simulink model "IEEE123_4subsystem"  (R2022b)
settings: Solver=ode4  StartTime=0.0  StopTime=inf  FixedStep=Ts  MaxStep=1e-4  RelTol=1e-3
PreLoadFcn:
  | Ts = 50e-6;
PostLoadFcn:
  | Ts = 50e-6;
InitFcn:
  | %%%%%%%%%%%%%%%%%%%%%%%%
  | % Simulation data for the IEEE 123 Node Test Feeder model
  | %%%%%%%%%%%%%%%%%%%%%%%
  | 
  | % miles/km
  | mi2km = 1.60934;
  | 
  | % feet to km
  | ft2km = 0.0003048;
  | 
  | % microsiemens to Farads
  | ms2F = 1/2/pi/60*1e-6;
  | 
  | %% Configuration 1 - series reactance - ohm/mile
  | 
  | R_1 = [0.4576 0.1560 0.1535;0.1560 0.4666 0.1580;0.1535 0.1580 0.4615];
  | X_1 = [1.0780 0.5017 0.3849;0.5017 1.0482 0.4236;0.3849 0.4236 1.0651];
  | 
  | % charging susceptance - microsiemens/mile
  | 
  | B_1 = [5.6765 -1.8319 -0.6982;-1.8319 5.9809 -1.1645;-0.6982 -1.1645 5.3971];
  | 
  | % convert for SPS
  | 
  | R_1 = R_1/mi2km;
  | 
  | Rs_1=(R_1(1,1)+R_1(2,2)+R_1(3,3))/3;
  | Rm_1=(R_1(1,2)+R_1(1,3)+R_1(2,3))/3;
  | R1_1=Rs_1-Rm_1;
  | R0_1=Rs_1+2*Rm_1;
  | 
  | L_1 = X_1/mi2km/2/pi/60;
  | 
  | Ls_1=(L_1(1,1)+L_1(2,2)+L_1(3,3))/3;
  | Lm_1=(L_1(1,2)+L_1(1,3)+L_1(2,3))/3;
  | L1_1=Ls_1-Lm_1;
  | L0_1=Ls_1+2*Lm_1;
  | 
  | C_1 = B_1/mi2km*ms2F;
  | 
  | Cs_1=(C_1(1,1)+C_1(2,2)+C_1(3,3))/3;
  | Cm_1=(C_1(1,2)+C_1(1,3)+C_1(2,3))/3;
  | C1_1=Cs_1-Cm_1;
  | C0_1=Cs_1+2*Cm_1;
  | 
  | 
  | %% Configuration 2 - series reactance - ohm/mile
  | 
  | R_2 = [0.4666 0.1580 0.1560;0.1580 0.4615 0.1535;0.1560 0.1535 0.4576];
  | X_2 = [1.0482 0.4236 0.5017;0.4236 1.0651 0.3849;0.5017 0.3849 1.0780];
  | 
  | % charging susceptance - microsiemens/mile
  | 
  | B_2 = [5.9809 -1.1645 -1.8319;-1.1645 5.3971 -0.6982;-1.8319 -0.6982 5.6765];
  | 
  | % convert for SPS
  | 
  | R_2 = R_2/mi2km;
  | 
  | Rs_2=(R_2(1,1)+R_2(2,2)+R_2(3,3))/3;
  | ... (+341 lines)
undefined symbols (not defined in the file): D1, Delta, find_system, I, Left, MOV_segment9, powergui, Right, type, V, X
libraries: spsGroundLib x242, spsThreePhaseVIMeasurementLib x134, spsSeriesRLCBranchLib x107, spsSeriesRLCLoadLib x83, spsPiSectionLineLib x61, spsThreePhasePISectionLineLib x60, spsVoltageMeasurementLib x52, spsDCVoltageSourceLib x36, ssn_lib x28, artemis x24, spsACCurrentSourceLib x18, spsOnDelayLib x18
(part 2 of 15)

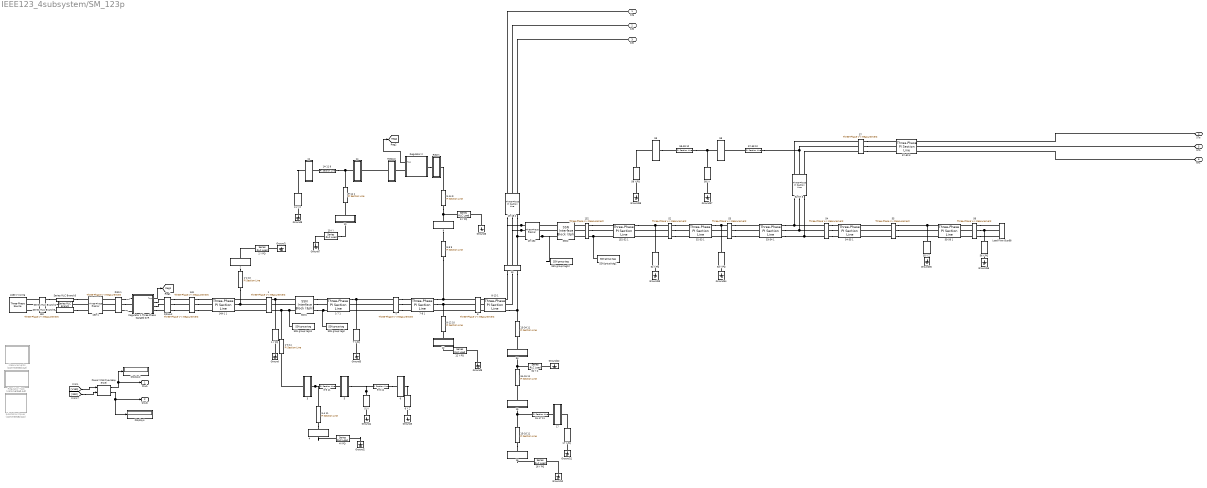
== system IEEE123_4subsystem/SM_123p ==
  1 : spsThreePhaseVIMeasurementLib/Three-Phase V-I Measurement  VoltageMeasurement=phase-to-ground  SetLabelV=on  LabelV=V1  Vpu=off  VpuLL=off  CurrentMeasurement=no  SetLabelI=on  LabelI=I800  Ipu=off  Pbase=100e6  Vbase=24900  OutputType=Complex  PhasorSimulation=off  PSBequivalent=0
  1 Y PQ : spsSeriesRLCLoadLib/Series RLC Load  LConnTagsString=a  RConnTagsString=__new0  NominalVoltage=1.0*2401.78  NominalFrequency=60  ActivePower=40e3  InductivePower=20e3  CapacitivePower=0  Setx0=off  InitialVoltage=0  SetiL0=off  InitialCurrent=0  Measurements=None  LoadType=constant PQ
  1-2 10 : spsPiSectionLineLib/Pi Section Line  LConnTagsString=__new0  RConnTagsString=__new0  Phases=1  PiSections=1  Length=175*ft2km  Frequency=60  Resistance=R1_10  Inductance=L1_10  Capacitance=C1_10  SpecifyConductance=off  Conductance=0  Measurements=None  Measurements2=None
      settings: LibrarySourceBlock=sps_lib/Power Grid Elements/Pi Section Line
  1-3 11 : spsPiSectionLineLib/Pi Section Line  LConnTagsString=__new0  RConnTagsString=__new0  Phases=1  PiSections=1  Length=250*ft2km  Frequency=60  Resistance=R1_11  Inductance=L1_11  Capacitance=C1_11  SpecifyConductance=off  Conductance=0  Measurements=None  Measurements2=None
      settings: LibrarySourceBlock=sps_lib/Power Grid Elements/Pi Section Line
  1-7 1 : spsThreePhasePISectionLineLib/Three-Phase PI Section Line  LConnTagsString=a|b|c  RConnTagsString=A|B|C  Length=300*ft2km  Frequency=60  Resistances=[R1_1 R0_1]  Inductances=[L1_1 L0_1]  Capacitances=[C1_1 C0_1]
  10 : Subsystem
  10 Y I : spsSeriesRLCLoadLib/Series RLC Load  LConnTagsString=a  RConnTagsString=__new0  NominalVoltage=1.0*2401.78  NominalFrequency=60  ActivePower=20e3  InductivePower=10e3  CapacitivePower=0  Setx0=off  InitialVoltage=0  SetiL0=off  InitialCurrent=0  Measurements=None  LoadType=constant I
  11 : Subsystem
  11 Y Z : spsSeriesRLCLoadLib/Series RLC Load  LConnTagsString=a  RConnTagsString=__new0  NominalVoltage=1.0*2401.78  NominalFrequency=60  ActivePower=40e3  InductivePower=20e3  CapacitivePower=0  Setx0=off  InitialVoltage=0  SetiL0=off  InitialCurrent=0  Measurements=None  LoadType=constant Z
  12 : Subsystem
  12 Y PQ : spsSeriesRLCLoadLib/Series RLC Load  LConnTagsString=a  RConnTagsString=__new0  NominalVoltage=1.0*2401.78  NominalFrequency=60  ActivePower=20e3  InductivePower=10e3  CapacitivePower=0  Setx0=off  InitialVoltage=0  SetiL0=off  InitialCurrent=0  Measurements=None  LoadType=constant PQ
  13 : spsThreePhaseVIMeasurementLib/Three-Phase V-I Measurement  VoltageMeasurement=phase-to-ground  SetLabelV=on  LabelV=V13  Vpu=off  VpuLL=off  CurrentMeasurement=yes  SetLabelI=on  LabelI=I13  Ipu=off  Pbase=100e6  Vbase=24900  OutputType=Complex  PhasorSimulation=off  PSBequivalent=0
  13-152 : spsThreePhaseBreakerLib/Three-Phase Breaker  InitialState=closed  SwitchA=on  SwitchB=on  SwitchC=on  SwitchTimes="[1/60  5/60]"  External=off  BreakerResistance=0.01  SnubberResistance=1e6  SnubberCapacitance=inf  Measurements=None
  13-18 2 : spsThreePhasePISectionLineLib/Three-Phase PI Section Line  LConnTagsString=a|b|c  RConnTagsString=A|B|C  Length=825*ft2km  Frequency=60  Resistances=[R1_2 R0_2]  Inductances=[L1_2 L0_2]  Capacitances=[C1_2 C0_2]
  13-34 11 : spsPiSectionLineLib/Pi Section Line  LConnTagsString=__new0  RConnTagsString=__new0  Phases=1  PiSections=1  Length=150*ft2km  Frequency=60  Resistance=R1_11  Inductance=L1_11  Capacitance=C1_11  SpecifyConductance=off  Conductance=0  Measurements=None  Measurements2=None
      settings: LibrarySourceBlock=sps_lib/Power Grid Elements/Pi Section Line
  14 : Subsystem
  14-11 9 : spsPiSectionLineLib/Pi Section Line  LConnTagsString=__new0  RConnTagsString=__new0  Phases=1  PiSections=1  Length=250*ft2km  Frequency=60  Resistance=R1_9  Inductance=L1_9  Capacitance=C1_9  SpecifyConductance=off  Conductance=0  Measurements=None  Measurements2=None
      settings: LibrarySourceBlock=sps_lib/Power Grid Elements/Pi Section Line
  149 : spsThreePhaseVIMeasurementLib/Three-Phase V-I Measurement  VoltageMeasurement=phase-to-ground  SetLabelV=on  LabelV=V149  Vpu=off  VpuLL=off  CurrentMeasurement=no  SetLabelI=on  LabelI=I800  Ipu=off  Pbase=100e6  Vbase=24900  OutputType=Complex  PhasorSimulation=off  PSBequivalent=0
  149-1 1 : spsThreePhasePISectionLineLib/Three-Phase PI Section Line  LConnTagsString=a|b|c  RConnTagsString=A|B|C  Length=400*ft2km  Frequency=60  Resistances=[R1_1 R0_1]  Inductances=[L1_1 L0_1]  Capacitances=[C1_1 C0_1]
  15 : Subsystem
  15-16 11 : spsPiSectionLineLib/Pi Section Line  LConnTagsString=__new0  RConnTagsString=__new0  Phases=1  PiSections=1  Length=375*ft2km  Frequency=60  Resistance=R1_11  Inductance=L1_11  Capacitance=C1_11  SpecifyConductance=off  Conductance=0  Measurements=None  Measurements2=None
      settings: LibrarySourceBlock=sps_lib/Power Grid Elements/Pi Section Line
  15-17 11 : spsPiSectionLineLib/Pi Section Line  LConnTagsString=__new0  RConnTagsString=__new0  Phases=1  PiSections=1  Length=350*ft2km  Frequency=60  Resistance=R1_11  Inductance=L1_11  Capacitance=C1_11  SpecifyConductance=off  Conductance=0  Measurements=None  Measurements2=None
      settings: LibrarySourceBlock=sps_lib/Power Grid Elements/Pi Section Line
  150 : spsThreePhaseVIMeasurementLib/Three-Phase V-I Measurement  VoltageMeasurement=phase-to-ground  SetLabelV=on  LabelV=V150  Vpu=off  VpuLL=off  CurrentMeasurement=yes  SetLabelI=on  LabelI=I150  Ipu=off  Pbase=100e6  Vbase=24900  OutputType=Complex  PhasorSimulation=off  PSBequivalent=0
  150-1 : spsThreePhaseBreakerLib/Three-Phase Breaker  InitialState=closed  SwitchA=on  SwitchB=on  SwitchC=on  SwitchTimes="[1/60  5/60]"  External=off  BreakerResistance=0.01  SnubberResistance=1e6  SnubberCapacitance=inf  Measurements=None
  152 : spsThreePhaseVIMeasurementLib/Three-Phase V-I Measurement  VoltageMeasurement=phase-to-ground  SetLabelV=on  LabelV=V152  Vpu=off  VpuLL=off  CurrentMeasurement=no  SetLabelI=on  LabelI=I65  Ipu=off  Pbase=100e6  Vbase=24900  OutputType=Complex  PhasorSimulation=off  PSBequivalent=0
  152-52 1 : spsThreePhasePISectionLineLib/Three-Phase PI Section Line  LConnTagsString=a|b|c  RConnTagsString=A|B|C  Length=400*ft2km  Frequency=60  Resistances=[R1_1 R0_1]  Inductances=[L1_1 L0_1]  Capacitances=[C1_1 C0_1]
  16 : Subsystem
  16 Y PQ : spsSeriesRLCLoadLib/Series RLC Load  LConnTagsString=a  RConnTagsString=__new0  NominalVoltage=1.0*2401.78  NominalFrequency=60  ActivePower=40e3  InductivePower=20e3  CapacitivePower=0  Setx0=off  InitialVoltage=0  SetiL0=off  InitialCurrent=0  Measurements=None  LoadType=constant PQ
  17 : Subsystem
  17 Y PQ : spsSeriesRLCLoadLib/Series RLC Load  LConnTagsString=a  RConnTagsString=__new0  NominalVoltage=1.0*2401.78  NominalFrequency=60  ActivePower=20e3  InductivePower=10e3  CapacitivePower=0  Setx0=off  InitialVoltage=0  SetiL0=off  InitialCurrent=0  Measurements=None  LoadType=constant PQ
  2 : Subsystem
  2 Y PQ : spsSeriesRLCLoadLib/Series RLC Load  LConnTagsString=a  RConnTagsString=__new0  NominalVoltage=1.0*2401.78  NominalFrequency=60  ActivePower=20e3  InductivePower=10e3  CapacitivePower=0  Setx0=off  InitialVoltage=0  SetiL0=off  InitialCurrent=0  Measurements=None  LoadType=constant PQ
  3 : Subsystem
  3-4 11 : spsPiSectionLineLib/Pi Section Line  LConnTagsString=__new0  RConnTagsString=__new0  Phases=1  PiSections=1  Length=200*ft2km  Frequency=60  Resistance=R1_11  Inductance=L1_11  Capacitance=C1_11  SpecifyConductance=off  Conductance=0  Measurements=None  Measurements2=None
      settings: LibrarySourceBlock=sps_lib/Power Grid Elements/Pi Section Line
  3-5 11 : spsPiSectionLineLib/Pi Section Line  LConnTagsString=__new0  RConnTagsString=__new0  Phases=1  PiSections=1  Length=325*ft2km  Frequency=60  Resistance=R1_11  Inductance=L1_11  Capacitance=C1_11  SpecifyConductance=off  Conductance=0  Measurements=None  Measurements2=None
      settings: LibrarySourceBlock=sps_lib/Power Grid Elements/Pi Section Line
  34 : Subsystem
  34 Y Z : spsSeriesRLCLoadLib/Series RLC Load  LConnTagsString=a  RConnTagsString=__new0  NominalVoltage=1.0*2401.78  NominalFrequency=60  ActivePower=40e3  InductivePower=20e3  CapacitivePower=0  Setx0=off  InitialVoltage=0  SetiL0=off  InitialCurrent=0  Measurements=None  LoadType=constant Z
  34-15 11 : spsPiSectionLineLib/Pi Section Line  LConnTagsString=__new0  RConnTagsString=__new0  Phases=1  PiSections=1  Length=100*ft2km  Frequency=60  Resistance=R1_11  Inductance=L1_11  Capacitance=C1_11  SpecifyConductance=off  Conductance=0  Measurements=None  Measurements2=None
      settings: LibrarySourceBlock=sps_lib/Power Grid Elements/Pi Section Line
  4 : Subsystem
  4160 V swing : spsThreePhaseSourceLib/Three-Phase Source  InternalConnection=Yg  VoltagePhases=on  Voltage=120e3  PhaseAngle=0  Voltage_phases=[1.0 1.0 1.0]*4160/sqrt(3)  PhaseAngles_phases=[0 -120 120 ]  Frequency=60  NonIdealSource=off  SpecifyImpedance=off  Resistance=.001  Inductance=16.58e-3  ShortCircuitLevel=100e6  BaseVoltage=4160  XRratio=10  BusType=swing  Pref=0  Qref=0  Prefabc=[0 0 0]  Qrefabc=[0 0 0]  Qmin="[-inf  -inf -inf]"  Qmax="[inf  inf inf]"
  4Y PQ : spsSeriesRLCLoadLib/Series RLC Load  LConnTagsString=a  RConnTagsString=__new0  NominalVoltage=1.0*2401.78  NominalFrequency=60  ActivePower=40e3  InductivePower=20e3  CapacitivePower=0  Setx0=off  InitialVoltage=0  SetiL0=off  InitialCurrent=0  Measurements=None  LoadType=constant PQ
  5 : Subsystem
  5 Y I : spsSeriesRLCLoadLib/Series RLC Load  LConnTagsString=a  RConnTagsString=__new0  NominalVoltage=1.0*2401.78  NominalFrequency=60  ActivePower=20e3  InductivePower=10e3  CapacitivePower=0  Setx0=off  InitialVoltage=0  SetiL0=off  InitialCurrent=0  Measurements=None  LoadType=constant I
  5-6 11 : spsPiSectionLineLib/Pi Section Line  LConnTagsString=__new0  RConnTagsString=__new0  Phases=1  PiSections=1  Length=250*ft2km  Frequency=60  Resistance=R1_11  Inductance=L1_11  Capacitance=C1_11  SpecifyConductance=off  Conductance=0  Measurements=None  Measurements2=None
      settings: LibrarySourceBlock=sps_lib/Power Grid Elements/Pi Section Line
  52 : spsThreePhaseVIMeasurementLib/Three-Phase V-I Measurement  VoltageMeasurement=phase-to-ground  SetLabelV=on  LabelV=V52  Vpu=off  VpuLL=off  CurrentMeasurement=yes  SetLabelI=on  LabelI=I52  Ipu=off  Pbase=100e6  Vbase=24900  OutputType=Complex  PhasorSimulation=off  PSBequivalent=0
  52 Y PQ : spsSeriesRLCLoadLib/Series RLC Load  LConnTagsString=a  RConnTagsString=__new0  NominalVoltage=1.0*2401.78  NominalFrequency=60  ActivePower=40e3  InductivePower=20e3  CapacitivePower=0  Setx0=off  InitialVoltage=0  SetiL0=off  InitialCurrent=0  Measurements=None  LoadType=constant PQ
  52-53 1 : spsThreePhasePISectionLineLib/Three-Phase PI Section Line  LConnTagsString=a|b|c  RConnTagsString=A|B|C  Length=200*ft2km  Frequency=60  Resistances=[R1_1 R0_1]  Inductances=[L1_1 L0_1]  Capacitances=[C1_1 C0_1]
  53 : spsThreePhaseVIMeasurementLib/Three-Phase V-I Measurement  VoltageMeasurement=phase-to-ground  SetLabelV=on  LabelV=V53  Vpu=off  VpuLL=off  CurrentMeasurement=no  SetLabelI=on  LabelI=I65  Ipu=off  Pbase=100e6  Vbase=24900  OutputType=Complex  PhasorSimulation=off  PSBequivalent=0
  53 Y PQ : spsSeriesRLCLoadLib/Series RLC Load  LConnTagsString=a  RConnTagsString=__new0  NominalVoltage=1.0*2401.78  NominalFrequency=60  ActivePower=40e3  InductivePower=20e3  CapacitivePower=0  Setx0=off  InitialVoltage=0  SetiL0=off  InitialCurrent=0  Measurements=None  LoadType=constant PQ
  53-54 1 : spsThreePhasePISectionLineLib/Three-Phase PI Section Line  LConnTagsString=a|b|c  RConnTagsString=A|B|C  Length=125*ft2km  Frequency=60  Resistances=[R1_1 R0_1]  Inductances=[L1_1 L0_1]  Capacitances=[C1_1 C0_1]
  54 : spsThreePhaseVIMeasurementLib/Three-Phase V-I Measurement  VoltageMeasurement=phase-to-ground  SetLabelV=on  LabelV=V54  Vpu=off  VpuLL=off  CurrentMeasurement=no  SetLabelI=on  LabelI=I65  Ipu=off  Pbase=100e6  Vbase=24900  OutputType=Complex  PhasorSimulation=off  PSBequivalent=0
  54-55 1 : spsThreePhasePISectionLineLib/Three-Phase PI Section Line  LConnTagsString=a|b|c  RConnTagsString=A|B|C  Length=275*ft2km  Frequency=60  Resistances=[R1_1 R0_1]  Inductances=[L1_1 L0_1]  Capacitances=[C1_1 C0_1]
  54-57 3 : spsThreePhasePISectionLineLib/Three-Phase PI Section Line  LConnTagsString=a|b|c  RConnTagsString=A|B|C  Length=350*ft2km  Frequency=60  Resistances=[R1_3 R0_3]  Inductances=[L1_3 L0_3]  Capacitances=[C1_3 C0_3]
  55 : spsThreePhaseVIMeasurementLib/Three-Phase V-I Measurement  VoltageMeasurement=phase-to-ground  SetLabelV=on  LabelV=V55  Vpu=off  VpuLL=off  CurrentMeasurement=no  SetLabelI=on  LabelI=I65  Ipu=off  Pbase=100e6  Vbase=24900  OutputType=Complex  PhasorSimulation=off  PSBequivalent=0
  55 Y Z : spsSeriesRLCLoadLib/Series RLC Load  LConnTagsString=a  RConnTagsString=__new0  NominalVoltage=1.0*2401.78  NominalFrequency=60  ActivePower=20e3  InductivePower=10e3  CapacitivePower=0  Setx0=off  InitialVoltage=0  SetiL0=off  InitialCurrent=0  Measurements=None  LoadType=constant Z
  55-56 1 : spsThreePhasePISectionLineLib/Three-Phase PI Section Line  LConnTagsString=a|b|c  RConnTagsString=A|B|C  Length=275*ft2km  Frequency=60  Resistances=[R1_1 R0_1]  Inductances=[L1_1 L0_1]  Capacitances=[C1_1 C0_1]
  56 : spsThreePhaseVIMeasurementLib/Three-Phase V-I Measurement  VoltageMeasurement=phase-to-ground  SetLabelV=on  LabelV=V56  Vpu=off  VpuLL=off  CurrentMeasurement=no  SetLabelI=on  LabelI=I65  Ipu=off  Pbase=100e6  Vbase=24900  OutputType=Complex  PhasorSimulation=off  PSBequivalent=0
  56 Y PQ : spsSeriesRLCLoadLib/Series RLC Load  LConnTagsString=a  RConnTagsString=__new0  NominalVoltage=1.0*2401.78  NominalFrequency=60  ActivePower=20e3  InductivePower=10e3  CapacitivePower=0  Setx0=off  InitialVoltage=0  SetiL0=off  InitialCurrent=0  Measurements=None  LoadType=constant PQ
  57 : spsThreePhaseVIMeasurementLib/Three-Phase V-I Measurement  VoltageMeasurement=phase-to-ground  SetLabelV=on  LabelV=V57  Vpu=off  VpuLL=off  CurrentMeasurement=no  SetLabelI=on  LabelI=I65  Ipu=off  Pbase=100e6  Vbase=24900  OutputType=Complex  PhasorSimulation=off  PSBequivalent=0
  57-58 10 : spsPiSectionLineLib/Pi Section Line  LConnTagsString=__new0  RConnTagsString=__new0  Phases=1  PiSections=1  Length=250*ft2km  Frequency=60  Resistance=R1_10  Inductance=L1_10  Capacitance=C1_10  SpecifyConductance=off  Conductance=0  Measurements=None  Measurements2=None
      settings: LibrarySourceBlock=sps_lib/Power Grid Elements/Pi Section Line
  57-60 3 : spsThreePhasePISectionLineLib/Three-Phase PI Section Line  LConnTagsString=a|b|c  RConnTagsString=A|B|C  Length=750*ft2km  Frequency=60  Resistances=[R1_3 R0_3]  Inductances=[L1_3 L0_3]  Capacitances=[C1_3 C0_3]
  58 : Subsystem
  58 Y I : spsSeriesRLCLoadLib/Series RLC Load  LConnTagsString=a  RConnTagsString=__new0  NominalVoltage=1.0*2401.78  NominalFrequency=60  ActivePower=20e3  InductivePower=10e3  CapacitivePower=0  Setx0=off  InitialVoltage=0  SetiL0=off  InitialCurrent=0  Measurements=None  LoadType=constant I
  58 Y PQ : spsSeriesRLCLoadLib/Series RLC Load  LConnTagsString=a  RConnTagsString=__new0  NominalVoltage=1.0*2401.78  NominalFrequency=60  ActivePower=20e3  InductivePower=10e3  CapacitivePower=0  Setx0=off  InitialVoltage=0  SetiL0=off  InitialCurrent=0  Measurements=None  LoadType=constant PQ
  58-59 10 : spsPiSectionLineLib/Pi Section Line  LConnTagsString=__new0  RConnTagsString=__new0  Phases=1  PiSections=1  Length=10*ft2km  Frequency=60  Resistance=R1_10  Inductance=L1_10  Capacitance=C1_10  SpecifyConductance=off  Conductance=0  Measurements=None  Measurements2=None
      settings: LibrarySourceBlock=sps_lib/Power Grid Elements/Pi Section Line
  59 : Subsystem
  6 : Subsystem
  6 Y Z : spsSeriesRLCLoadLib/Series RLC Load  LConnTagsString=a  RConnTagsString=__new0  NominalVoltage=1.0*2401.78  NominalFrequency=60  ActivePower=40e3  InductivePower=20e3  CapacitivePower=0  Setx0=off  InitialVoltage=0  SetiL0=off  InitialCurrent=0  Measurements=None  LoadType=constant Z
  7 : spsThreePhaseVIMeasurementLib/Three-Phase V-I Measurement  VoltageMeasurement=phase-to-ground  SetLabelV=on  LabelV=V7  Vpu=off  VpuLL=off  CurrentMeasurement=no  SetLabelI=on  LabelI=I800  Ipu=off  Pbase=100e6  Vbase=24900  OutputType=Complex  PhasorSimulation=off  PSBequivalent=0
  7 Y PQ : spsSeriesRLCLoadLib/Series RLC Load  LConnTagsString=a  RConnTagsString=__new0  NominalVoltage=1.0*2401.78  NominalFrequency=60  ActivePower=20e3  InductivePower=10e3  CapacitivePower=0  Setx0=off  InitialVoltage=0  SetiL0=off  InitialCurrent=0  Measurements=None  LoadType=constant PQ
  7-8 1 : spsThreePhasePISectionLineLib/Three-Phase PI Section Line  LConnTagsString=a|b|c  RConnTagsString=A|B|C  Length=200*ft2km  Frequency=60  Resistances=[R1_1 R0_1]  Inductances=[L1_1 L0_1]  Capacitances=[C1_1 C0_1]
  8 : spsThreePhaseVIMeasurementLib/Three-Phase V-I Measurement  VoltageMeasurement=phase-to-ground  SetLabelV=on  LabelV=V8  Vpu=off  VpuLL=off  CurrentMeasurement=no  SetLabelI=on  LabelI=I800  Ipu=off  Pbase=100e6  Vbase=24900  OutputType=Complex  PhasorSimulation=off  PSBequivalent=0
  8-12 10 : spsPiSectionLineLib/Pi Section Line  LConnTagsString=__new0  RConnTagsString=__new0  Phases=1  PiSections=1  Length=225*ft2km  Frequency=60  Resistance=R1_10  Inductance=L1_10  Capacitance=C1_10  SpecifyConductance=off  Conductance=0  Measurements=None  Measurements2=None
      settings: LibrarySourceBlock=sps_lib/Power Grid Elements/Pi Section Line
  8-13 1 : spsThreePhasePISectionLineLib/Three-Phase PI Section Line  LConnTagsString=a|b|c  RConnTagsString=A|B|C  Length=300*ft2km  Frequency=60  Resistances=[R1_1 R0_1]  Inductances=[L1_1 L0_1]  Capacitances=[C1_1 C0_1]
  8-9 9 : spsPiSectionLineLib/Pi Section Line  LConnTagsString=__new0  RConnTagsString=__new0  Phases=1  PiSections=1  Length=225*ft2km  Frequency=60  Resistance=R1_9  Inductance=L1_9  Capacitance=C1_9  SpecifyConductance=off  Conductance=0  Measurements=None  Measurements2=None
      settings: LibrarySourceBlock=sps_lib/Power Grid Elements/Pi Section Line
  9 : Subsystem
  9 Y PQ : spsSeriesRLCLoadLib/Series RLC Load  LConnTagsString=a  RConnTagsString=__new0  NominalVoltage=1.0*2401.78  NominalFrequency=60  ActivePower=40e3  InductivePower=20e3  CapacitivePower=0  Setx0=off  InitialVoltage=0  SetiL0=off  InitialCurrent=0  Measurements=None  LoadType=constant PQ
  9-14 1 : spsPiSectionLineLib/Pi Section Line  LConnTagsString=__new0  RConnTagsString=__new0  Phases=1  PiSections=1  Length=250*ft2km  Frequency=60  Resistance=R1_9  Inductance=L1_9  Capacitance=C1_9  SpecifyConductance=off  Conductance=0  Measurements=None  Measurements2=None
      settings: LibrarySourceBlock=sps_lib/Power Grid Elements/Pi Section Line
  9-14 9 : spsPiSectionLineLib/Pi Section Line  LConnTagsString=__new0  RConnTagsString=__new0  Phases=1  PiSections=1  Length=425*ft2km  Frequency=60  Resistance=R1_9  Inductance=L1_9  Capacitance=C1_9  SpecifyConductance=off  Conductance=0  Measurements=None  Measurements2=None
      settings: LibrarySourceBlock=sps_lib/Power Grid Elements/Pi Section Line
  Display2 : Display
  Display4 : Display
  Ground{,1..11,22,33..38} (19 alike) : spsGroundLib/Ground  LConnTagsString=a
  Load Flow Bus68 : spsLoadFlowBusLib/Load Flow Bus  LConnTagsString=a|b|c  Phases=ABC  Connectors=on one side  ID=56  Vbase=4160/sqrt(3)  Vref=[1.0 1.0 1.0]  Vangle=[0 -120 120]  VLF=1  VLFb=1  VLFc=1  angleLF=0  angleLFb=0  angleLFc=0
  Measurements : Subsystem  Commented=on
  Power (Positive-Sequence) : spsPowerPositiveSequenceLib/Power (Positive-Sequence)  Freq=60  Vinit=[0, 0]  Iinit=[0, 0]  Ts=Ts
      settings: LibrarySourceBlock=|
      | sps_lib/Sensors and Measurements/Power
      | (Positive-Sequence)
  RG1in : spsThreePhaseVIMeasurementLib/Three-Phase V-I Measurement  VoltageMeasurement=phase-to-ground  SetLabelV=on  LabelV=RG1in  Vpu=off  VpuLL=off  CurrentMeasurement=no  SetLabelI=on  LabelI=I800  Ipu=off  Pbase=100e6  Vbase=24900  OutputType=Complex  PhasorSimulation=off  PSBequivalent=0
  RG1out : spsThreePhaseVIMeasurementLib/Three-Phase V-I Measurement  VoltageMeasurement=phase-to-ground  SetLabelV=on  LabelV=RG1out  Vpu=off  VpuLL=off  CurrentMeasurement=no  SetLabelI=on  LabelI=I800  Ipu=off  Pbase=100e6  Vbase=24900  OutputType=Complex  PhasorSimulation=off  PSBequivalent=0
  RG2in : Subsystem
  RG2out : Subsystem
  Regulator 1 Three Phase Ganged SVR : Subsystem
  Regulator 2 : Subsystem
  Regulator Taps : Subsystem  Commented=on
  SSN group tag1 : artemis/SSN/SSN group tag  ssn_group_tag=ssn2b
  SSN group tag11 : artemis/SSN/SSN group tag  ssn_group_tag=ssn1a
  SSN group tag12 : artemis/SSN/SSN group tag  ssn_group_tag=ssn2a
  SSN group tag2 : artemis/SSN/SSN group tag  ssn_group_tag=ssn1b
  SSN1 : ssn_lib/SSN Interface Block (3ph)  nb_phase=3  nb_port=2  p1_type=I-type(Left)  p2_type=I-type(Right)  p3_type=V-type(Left)  p4_type=V-type(Left)  p5_type=V-type(Left)  p6_type=V-type(Left)  p7_type=V-type(Left)  p8_type=V-type(Left)  p9_type=V-type(Left)  p10_type=V-type(Left)  p11_type=V-type(Left)  p12_type=V-type(Left)  p13_type=V-type(Left)  p14_type=V-type(Left)  p15_type=V-type(Left)  p16_type=V-type(Left)  I_port_shunt_resistance=1e9
  SSN2 : ssn_lib/SSN Interface Block (3ph)  nb_phase=3  nb_port=2  p1_type=I-type(Left)  p2_type=I-type(Right)  p3_type=V-type(Left)  p4_type=V-type(Left)  p5_type=V-type(Left)  p6_type=V-type(Left)  p7_type=V-type(Left)  p8_type=V-type(Left)  p9_type=V-type(Left)  p10_type=V-type(Left)  p11_type=V-type(Left)  p12_type=V-type(Left)  p13_type=V-type(Left)  p14_type=V-type(Left)  p15_type=V-type(Left)  p16_type=V-type(Left)  I_port_shunt_resistance=1e9
  Series RLC Branch3 : spsSeriesRLCBranchLib/Series RLC Branch  LConnTagsString=__new0  RConnTagsString=__new0  BranchType=R  Resistance=.0001  Inductance=0  SetiL0=off  InitialCurrent=0  Capacitance=0  Setx0=off  InitialVoltage=0  Measurements=None
  Series RLC Branch4 : spsSeriesRLCBranchLib/Series RLC Branch  LConnTagsString=__new0  RConnTagsString=__new0  BranchType=R  Resistance=.0001  Inductance=0  SetiL0=off  InitialCurrent=0  Capacitance=0  Setx0=off  InitialVoltage=0  Measurements=None
  Series RLC Branch5 : spsSeriesRLCBranchLib/Series RLC Branch  LConnTagsString=__new0  RConnTagsString=__new0  BranchType=R  Resistance=.0001  Inductance=0  SetiL0=off  InitialCurrent=0  Capacitance=0  Setx0=off  InitialVoltage=0  Measurements=None
  Substation Power : Subsystem  Commented=on
  13a : PMIOPort  Side=Right
  13b : PMIOPort  Port=2  Side=Right
  13c : PMIOPort  Port=3  Side=Right
  57a : PMIOPort  Port=4  Side=Right
  57b : PMIOPort  Port=5  Side=Right
  57c : PMIOPort  Port=6  Side=Right
  Psub : Outport
  Qsub : Outport  Port=2
  tag scope: Reg1=global, Reg2=global
  wires:
  [V150] -> Power (Positive-Sequence)/1
  Power (Positive-Sequence)/1 -> Display2/1, Psub/1
  Power (Positive-Sequence)/2 -> Qsub/1, Display4/1
  [I150] -> Power (Positive-Sequence)/2
  Regulator 2/1(Tap) -> [Reg2]
  Regulator 1 Three Phase Ganged SVR/1(Tap) -> [Reg1]
  connections:
  8/LConn1 -- 8-9 9/LConn1 -- 7-8 1/RConn1
  54-57 3/LConn1 -- 54/LConn1 -- 53-54 1/RConn1
  Ground38/LConn1 -- 58 Y PQ/RConn1
  54-57 3/LConn3 -- 53-54 1/RConn3 -- 54/LConn3
  RG2out/RConn1 -- 14/LConn1
  34 Y Z/LConn1 -- 34-15 11/LConn1 -- 34/RConn1
  Ground22/LConn1 -- 34 Y Z/RConn1
  54-57 3/LConn2 -- 53-54 1/RConn2 -- 54/LConn2
  5 Y I/LConn1 -- 5-6 11/LConn1 -- 5/RConn1
  SSN group tag1/LConn1 -- 152-52 1/LConn3 -- 152/RConn3
  Ground11/LConn1 -- 17 Y PQ/RConn1
  13-152/LConn2 -- 13-18 2/LConn2 -- 13/RConn2
  14/RConn1 -- 14-11 9/LConn1 -- 9-14 1/LConn1
  13-152/LConn3 -- 13-18 2/LConn3 -- 13/RConn3
  11/RConn1 -- 11 Y Z/LConn1
  5/LConn1 -- 3-5 11/RConn1
  Ground36/LConn1 -- 56 Y PQ/RConn1
  8-13 1/RConn3 -- 13-34 11/LConn1 -- 13/LConn3
  5-6 11/RConn1 -- 6/LConn1
  52/LConn1 -- 52 Y PQ/LConn1 -- 152-52 1/RConn1
  150-1/LConn2 -- Series RLC Branch4/RConn1
  7/RConn3 -- 7-8 1/LConn3
  SSN2/LConn2 -- 13-152/RConn2
  149/RConn1 -- 149-1 1/LConn1
  8/LConn2 -- 8-12 10/LConn1 -- 7-8 1/RConn2
  RG1out/RConn2 -- 149/LConn2
  52/RConn1 -- 52-53 1/LConn1
  53/LConn1 -- 53 Y PQ/LConn1 -- 52-53 1/RConn1
  SSN1/LConn3 -- 1/RConn3 -- 1-3 11/LConn1 -- SSN group tag11/LConn1
  RG1in/LConn3 -- 150-1/RConn3
  53/RConn2 -- 53-54 1/LConn2
  53/RConn3 -- 53-54 1/LConn3
  56/RConn2 -- 56 Y PQ/LConn1 -- Load Flow Bus68/LConn2
  1/LConn1 -- 149-1 1/RConn1
  58/RConn1 -- 58 Y I/LConn1 -- 58-59 10/LConn1
  59/LConn1 -- 58-59 10/RConn1
  15-16 11/LConn1 -- 15-17 11/LConn1 -- 15/RConn1
  55/LConn1 -- 54-55 1/RConn1
  3-5 11/LConn1 -- 3-4 11/LConn1 -- 3/RConn1
  53/RConn1 -- 53-54 1/LConn1
  54-57 3/RConn2 -- 57/RConn2 -- 57-58 10/LConn1
  13-152/RConn3 -- SSN2/LConn3 -- SSN group tag12/LConn1
  7 Y PQ/LConn1 -- 1-7 1/RConn1 -- 7/LConn1
  152/RConn1 -- 152-52 1/LConn1
  1/LConn3 -- 149-1 1/RConn3
  150/RConn1 -- Series RLC Branch3/LConn1
  RG1out/RConn1 -- 149/LConn1
  57/RConn3 -- 54-57 3/RConn3
  9 Y PQ/LConn1 -- 9-14 9/LConn1 -- 9/RConn1
  150/LConn3 -- 4160 V swing/RConn3
  54/RConn3 -- 54-55 1/LConn3
  Ground37/LConn1 -- 58 Y I/RConn1
  57b/RConn1 -- 57-60 3/RConn2
  Ground33/LConn1 -- 52 Y PQ/RConn1
  55-56 1/LConn1 -- 55 Y Z/LConn1 -- 55/RConn1
  13-152/LConn1 -- 13-18 2/LConn1 -- 13/RConn1
  10 Y I/LConn1 -- 10/RConn1
  149-1 1/RConn2 -- 1/LConn2 -- 1-2 10/LConn1
  57/RConn1 -- 54-57 3/RConn1
  8/LConn3 -- 7-8 1/RConn3
  57/LConn3 -- 57-60 3/LConn3
  1-7 1/LConn3 -- SSN1/RConn3 -- SSN group tag2/LConn1
  17 Y PQ/LConn1 -- 17/RConn1
  1/RConn1 -- 1 Y PQ/LConn1 -- SSN1/LConn1
  54/RConn2 -- 54-55 1/LConn2
  55/LConn3 -- 54-55 1/RConn3
  54/RConn1 -- 54-55 1/LConn1
  RG2in/LConn1 -- 9-14 9/RConn1
  Regulator 1 Three Phase Ganged SVR/RConn2 -- RG1out/LConn2
  Ground8/LConn1 -- 11 Y Z/RConn1
  150/RConn2 -- Series RLC Branch4/LConn1
  Ground3/LConn1 -- 6 Y Z/RConn1
  12/LConn1 -- 8-12 10/RConn1
  52/LConn2 -- 152-52 1/RConn2
  Ground9/LConn1 -- 12 Y PQ/RConn1
  9/LConn1 -- 8-9 9/RConn1
  Ground34/LConn1 -- 53 Y PQ/RConn1
  55/RConn3 -- 55-56 1/LConn3
  Ground2/LConn1 -- 4Y PQ/RConn1
  150/RConn3 -- Series RLC Branch5/LConn1
  149/RConn3 -- 149-1 1/LConn3
  52/RConn3 -- 52-53 1/LConn3
  Regulator 1 Three Phase Ganged SVR/RConn1 -- RG1out/LConn1
  Ground35/LConn1 -- 55 Y Z/RConn1
  Ground5/LConn1 -- 7 Y PQ/RConn1
  3/LConn1 -- 1-3 11/RConn1
  Ground/LConn1 -- 1 Y PQ/RConn1
  Ground4/LConn1 -- 5 Y I/RConn1
  56/LConn3 -- 55-56 1/RConn3
  57-58 10/RConn1 -- 58/LConn1
  150/LConn1 -- 4160 V swing/RConn1
  Series RLC Branch5/RConn1 -- 150-1/LConn3
  150/LConn2 -- 4160 V swing/RConn2
  Ground6/LConn1 -- 9 Y PQ/RConn1
  7/RConn1 -- 7-8 1/LConn1
  34/LConn1 -- 13-34 11/RConn1
  2 Y PQ/LConn1 -- 2/RConn1
  53/LConn2 -- 52-53 1/RConn2
  52/RConn2 -- 52-53 1/LConn2
  4/RConn1 -- 4Y PQ/LConn1
  RG1out/RConn3 -- 149/LConn3
  149/RConn2 -- 149-1 1/LConn2
  Ground1/LConn1 -- 2 Y PQ/RConn1
  8/RConn1 -- 8-13 1/LConn1
  7/LConn3 -- 1-7 1/RConn3
  58 Y PQ/LConn1 -- 59/RConn1
  10/LConn1 -- 9-14 1/RConn1
  8/RConn3 -- 8-13 1/LConn3
  16/RConn1 -- 16 Y PQ/LConn1
  13/LConn1 -- 8-13 1/RConn1
  152/LConn3 -- SSN2/RConn3
  7/LConn2 -- 1-7 1/RConn2
  Ground10/LConn1 -- 16 Y PQ/RConn1
  52/LConn3 -- 152-52 1/RConn3
  3-4 11/RConn1 -- 4/LConn1
  13/LConn2 -- 8-13 1/RConn2
  SSN1/RConn1 -- 1-7 1/LConn1
  15-16 11/RConn1 -- 16/LConn1
  55/RConn2 -- 55-56 1/LConn2
  56/RConn3 -- Load Flow Bus68/LConn3
  Regulator 2/RConn1 -- RG2out/LConn1
  17/LConn1 -- 15-17 11/RConn1
  RG1in/RConn2 -- Regulator 1 Three Phase Ganged SVR/LConn2
  RG1in/RConn1 -- Regulator 1 Three Phase Ganged SVR/LConn1
  12 Y PQ/LConn1 -- 12/RConn1
  Ground7/LConn1 -- 10 Y I/RConn1
  152/LConn2 -- SSN2/RConn2
  8/RConn2 -- 8-13 1/LConn2
  SSN1/RConn2 -- 1-7 1/LConn2
  RG1in/LConn2 -- 150-1/RConn2
  1/RConn2 -- SSN1/LConn2
  Regulator 1 Three Phase Ganged SVR/LConn3 -- RG1in/RConn3
  55/LConn2 -- 54-55 1/RConn2
  7/RConn2 -- 7-8 1/LConn2
  2/LConn1 -- 1-2 10/RConn1
  14-11 9/RConn1 -- 11/LConn1
  6/RConn1 -- 6 Y Z/LConn1
  56/LConn2 -- 55-56 1/RConn2
  RG1in/LConn1 -- 150-1/RConn1
  152/LConn1 -- SSN2/RConn1
  56/RConn1 -- Load Flow Bus68/LConn1
  57/LConn1 -- 57-60 3/LConn1
  Series RLC Branch3/RConn1 -- 150-1/LConn1
  57/LConn2 -- 57-60 3/LConn2
  15/LConn1 -- 34-15 11/RConn1
  56/LConn1 -- 55-56 1/RConn1
  53/LConn3 -- 52-53 1/RConn3
  Regulator 2/LConn1 -- RG2in/RConn1
  152/RConn2 -- 152-52 1/LConn2
  SSN2/LConn1 -- 13-152/RConn1
  13c/RConn1 -- 13-18 2/RConn3
  57c/RConn1 -- 57-60 3/RConn3
  13a/RConn1 -- 13-18 2/RConn1
  13b/RConn1 -- 13-18 2/RConn2
  57a/RConn1 -- 57-60 3/RConn1
  Regulator 1 Three Phase Ganged SVR/RConn3 -- RG1out/LConn3
